simulink model "proj_ref"  (R2021b)
settings: Solver=VariableStepAuto  StartTime=0.0  StopTime=tf  RelTol=1e-3
values from neighbouring files (symbols this model uses):
  alpha_p = 10    [project_code_Nonlinear.m]
  beta_p = 10    [project_code_Nonlinear.m]
  k1 = (m*g*l)/(2*I)    (= 0.751533742331)    [project_code_Nonlinear.m]
  k2 = 1/I    (= 0.0766871165644)    [project_code_Nonlinear.m]
  theta_d = 10*init + (last+init)*randn(N,1)    [project_code_Nonlinear.m]
  x1_IC = init + (last+init)*randn(N,1)    [project_code_Nonlinear.m]
  x2_IC = init + (last+init)*randn(N,1)    [project_code_Nonlinear.m]
settings Model: Creator=kaush  LastModifiedBy=kaush

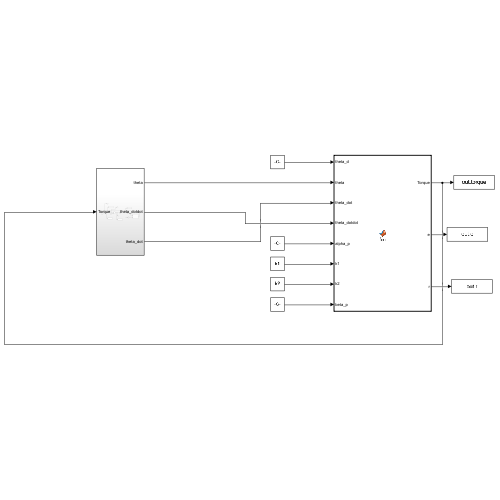
[thumbnail: Simulink's stored preview of the top-level diagram]
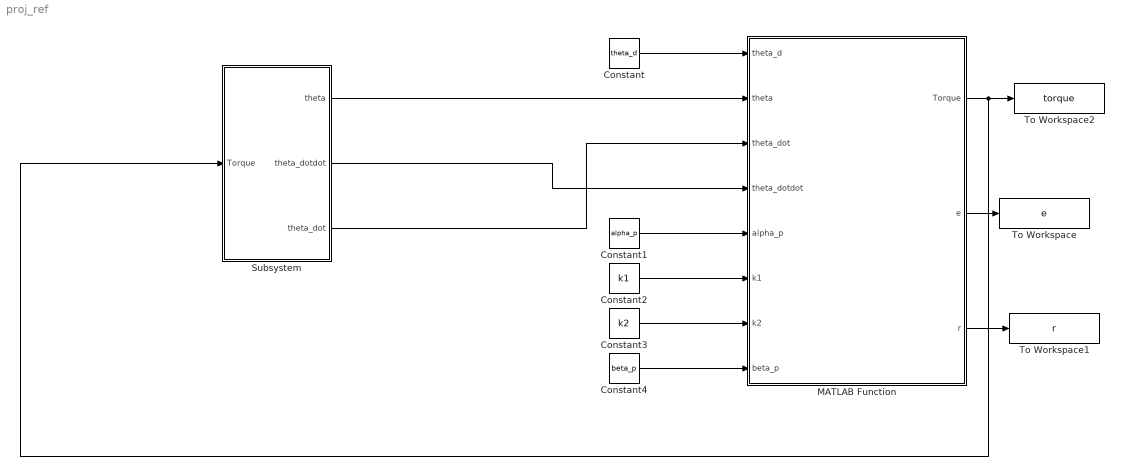
== system proj_ref ==
  Constant : Constant  Value=theta_d
  Constant1 : Constant  Value=alpha_p
  Constant2 : Constant  Value=k1
  Constant3 : Constant  Value=k2
  Constant4 : Constant  Value=beta_p
  MATLAB Function : MATLAB Function  TreatAsAtomicUnit=on
  Subsystem : Subsystem
  To Workspace : ToWorkspace  VariableName=e  SaveFormat=Timeseries  SampleTime=-1
  To Workspace1 : ToWorkspace  VariableName=r  SaveFormat=Timeseries  SampleTime=-1
  To Workspace2 : ToWorkspace  VariableName=torque  SaveFormat=Timeseries  SampleTime=-1
  wires:
  Subsystem/1(theta) -> MATLAB Function/2(theta)
  Subsystem/2(theta_dotdot) -> MATLAB Function/4(theta_dotdot)
  Subsystem/3(theta_dot) -> MATLAB Function/3(theta_dot)
  Constant/1 -> MATLAB Function/1(theta_d)
  Constant1/1 -> MATLAB Function/5(alpha_p)
  Constant2/1 -> MATLAB Function/6(k1)
  Constant3/1 -> MATLAB Function/7(k2)
  Constant4/1 -> MATLAB Function/8(beta_p)
  MATLAB Function/2(e) -> To Workspace/1
  MATLAB Function/3(r) -> To Workspace1/1
  MATLAB Function/1(Torque) -> Subsystem/1(Torque), To Workspace2/1

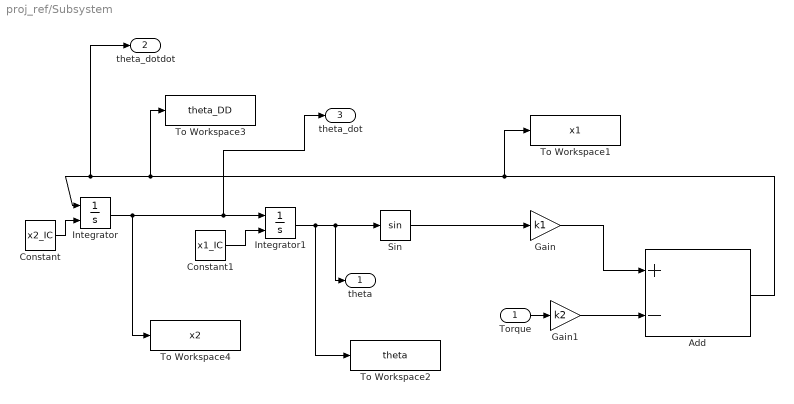
== system proj_ref/Subsystem ==
  Torque : Inport
  Add : Sum  Inputs=+-
  Constant : Constant  Value=x2_IC
  Constant1 : Constant  Value=x1_IC
  Gain : Gain  Gain=k1
  Gain1 : Gain  Gain=k2
  Integrator : Integrator  InitialConditionSource=external
  Integrator1 : Integrator  InitialConditionSource=external
  Sin : Trigonometry
  To Workspace1 : ToWorkspace  VariableName=x1  SaveFormat=Timeseries  SampleTime=-1
  To Workspace2 : ToWorkspace  VariableName=theta  SaveFormat=Timeseries  SampleTime=-1
  To Workspace3 : ToWorkspace  VariableName=theta_DD  SaveFormat=Timeseries  SampleTime=-1
  To Workspace4 : ToWorkspace  VariableName=x2  SaveFormat=Timeseries  SampleTime=-1
  theta : Outport
  theta_dotdot : Outport  Port=2
  theta_dot : Outport  Port=3
  wires:
  Integrator/1 -> To Workspace4/1, theta_dot/1, Integrator1/1
  Constant/1 -> Integrator/2
  Gain1/1 -> Add/2
  Sin/1 -> Gain/1
  Integrator1/1 -> To Workspace2/1, theta/1, Sin/1
  Add/1 -> To Workspace1/1, To Workspace3/1, theta_dotdot/1, Integrator/1
  Constant1/1 -> Integrator1/2
  Gain/1 -> Add/1
  Torque/1 -> Gain1/1

== matlab function proj_ref/MATLAB Function ==
  data: theta_d input; Torque output; theta input; theta_dot input; theta_dotdot input; alpha_p input; k1 input; k2 input; beta_p input; e output; r output
function [Torque, e, r]  = fcn(theta_d, theta, theta_dot, theta_dotdot, alpha_p, k1, k2, beta_p )
e = theta_d - theta;
e_dot = - theta_dot;
e_dotdot = - theta_dotdot;
r = e_dot + alpha_p*e;
r_dot = e_dotdot + alpha_p*e_dot;
Torque = (k1/k2)*sin(theta) - (alpha_p/k2)*e_dot - e - beta_p*r;
